simulink model "Aufgabe_3"  (R2023b)
settings: Solver=VariableStepAuto  StartTime=0.0  StopTime=4200  RelTol=1e-3
settings Model: Creator=danie  LastModifiedBy=danie

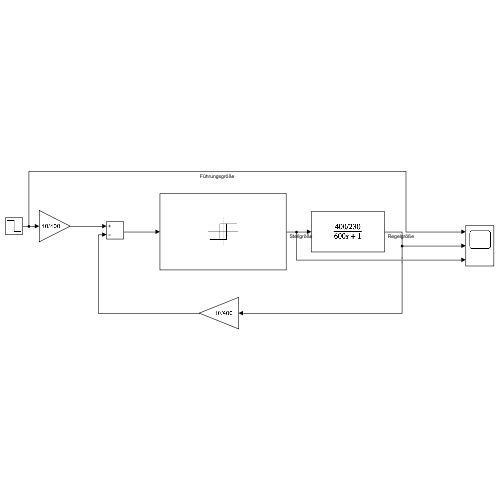
[thumbnail: Simulink's stored preview of the top-level diagram]
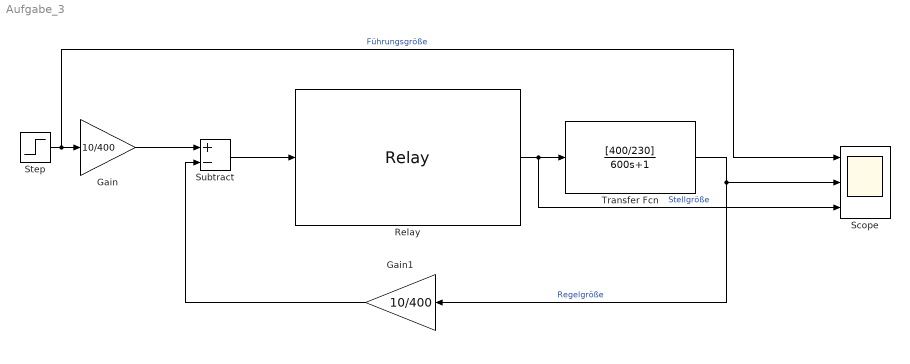
== system Aufgabe_3 ==
  Gain : Gain  Gain=10/400
  Gain1 : Gain  Gain=10/400
  Relay : Relay  OnSwitchValue=0.75  OffSwitchValue=-0.75  OnOutputValue=230
  Scope : Scope  NumInputPorts=3
  Step : Step  Time=1800  Before=180  After=0  SampleTime=0
  Subtract : Sum  Inputs=+-
  Transfer Fcn : TransferFcn  Numerator=[400/230]  Denominator=[600 1]
  wires:
  Gain/1 -> Subtract/1
  Subtract/1 -> Relay/1
  Relay/1 -> Scope/3, Transfer Fcn/1  "Stellgröße"
  Transfer Fcn/1 -> Scope/2, Gain1/1  "Regelgröße"
  Gain1/1 -> Subtract/2
  Step/1 -> Scope/1, Gain/1  "Führungsgröße"
